simulink model "Application_Problem_Solution"  (R2018b)
settings: Solver=VariableStepAuto  StartTime=0.0  StopTime=6300  FixedStep=0.1  RelTol=1e-3  EnableMultiTasking=on
StopFcn:
  | if sum(Diagnostic_Decision_PV_1)>0
  | f = msgbox('Failure in PV 1');
  | end
  | 
  | if sum(Diagnostic_Decision_PV_2)>0
  | f = msgbox('Failure in PV 2');
  | end
  | 
  | if sum(Diagnostic_Decision_PV_3)>0
  | f = msgbox('Failure in PV 3');
  | end
  | 
  | if sum(Diagnostic_Decision_PV_4)>0
  | f = msgbox('Failure in PV 4');
  | end
  | 
  | if sum(Diagnostic_Decision_PV_5)>0
  | f = msgbox('Failure in PV 5');
  | end
  | 
  | if sum(Diagnostic_Decision_PV_6)>0
  | f = msgbox('Failure in PV 6');
  | end
  | 
  | if sum(Diagnostic_Decision_PV_7)>0
  | f = msgbox('Failure in PV 7');
  | end
  | 
  | if sum(Diagnostic_Decision_PV_8)>0
  | f = msgbox('Failure in PV 8');
  | end
  | 
  | if sum(Diagnostic_Decision_PV_9)>0
  | f = msgbox('Failure in PV 9');
  | end
  | 
  | if sum(Diagnostic_Decision_PV_10)>0
  | f = msgbox('Failure in PV 10');
  | end
values from neighbouring files (symbols this model uses):
  C1_LUT = [1913.6 4625.7 23306 10736 18036 12251 9022.9 12447 18872 40764 18721 33630 ... (21 elements, 7x3)]    [model_data_application.mat]
  Capacity_LUT = [28.0081 27.625 27.6392]    [model_data_application.mat]
  cell_Cp_heat = 810.5328    [model_data_application.mat]
  cell_mass = 1    [model_data_application.mat]
  Em_LUT = [3.4966 3.5519 3.6183 3.7066 3.9131 4.0748 4.1923 3.5057 3.566 3.6337 3.7127 3.9259 ... (21 elements, 7x3)]    [model_data_application.mat]
  Qe_init = 3.6845    [model_data_application.mat]
  R0_LUT = [0.0117 0.011 0.0114 0.0107 0.0107 0.0113 0.0116 0.0085 0.0085 0.0087 0.0082 0.0083 ... (21 elements, 7x3)]    [model_data_application.mat]
  R1_LUT = [0.0109 0.0069 0.0047 0.0034 0.0033 0.0033 0.0028 0.0029 0.0024 0.0026 0.0016 0.0023 ... (21 elements, 7x3)]    [model_data_application.mat]
  SOC_LUT = [0 0.1 0.25 0.5 0.75 0.9 1]    [model_data_application.mat]
  T_init = 293.15    [model_data_application.mat]
  Temperature_LUT = [278.15 293.15 313.15]    [model_data_application.mat]
undefined symbols (not defined in the file or in its folder): DiscIntNeverNeededParam
libraries: elec_lib x450, fl_lib x121, LiBatteryElements_lib x40, nesl_utility x32, simulink x10
(part 3 of 3)

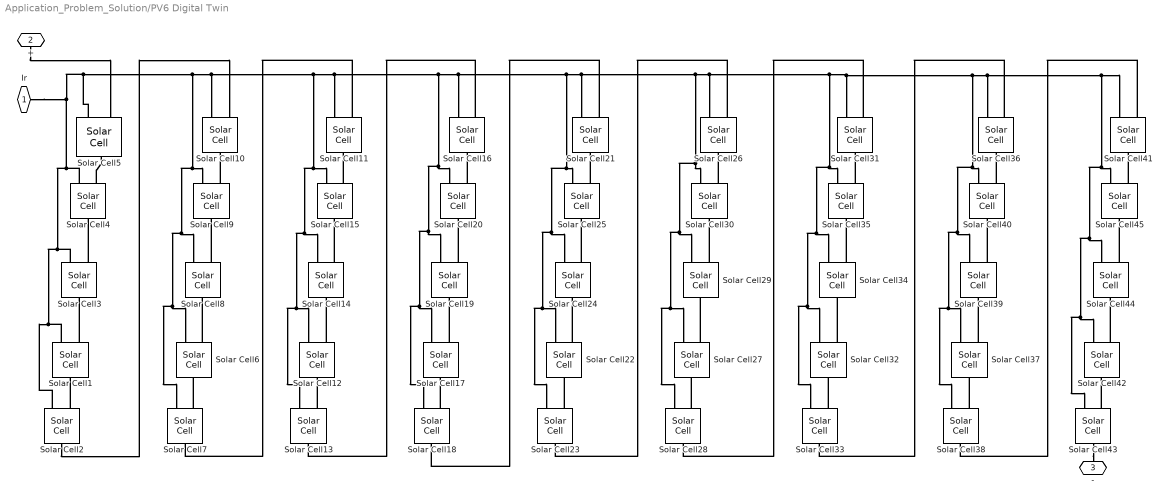
== system Application_Problem_Solution/PV6 Digital Twin ==
  Solar Cell{1..45} (45 alike) : elec_lib/Sources/Solar Cell  prm=1  Isc=Isc A  Voc=Voc/45 V  Is=1e-6 A  Is2=0 A  Iph=7.34 A  Ir0=Ir0 W/m^2  ec=n  N2=2  Rs=Rs/45 Ohm  Rp=Inf Ohm  N_series=1  TIPH1=0 1/K  EG=1.11 eV  TXIS1=3  TXIS2=3  TRS1=0  TRP1=0  Tmeas=T degC  TFIXED=T degC  thermal_mass=100 J/K  initial_temperature=25 degC
      settings: SourceProductName=Simscape Electronics  SourceProductBaseCode=SN
  Ir : PMIOPort  Side=Left
  + : PMIOPort  Port=2  Side=Right
  - : PMIOPort  Port=3  Side=Right
  connections:
  Solar Cell43/RConn1 -- -/RConn1
  Solar Cell43/LConn2 -- Solar Cell42/RConn1
  Solar Cell42/LConn2 -- Solar Cell44/RConn1
  Solar Cell45/LConn2 -- Solar Cell41/RConn1
  Solar Cell41/LConn2 -- Solar Cell38/RConn1
  Solar Cell44/LConn2 -- Solar Cell45/RConn1
  Solar Cell38/LConn2 -- Solar Cell37/RConn1
  Solar Cell37/LConn2 -- Solar Cell39/RConn1
  Solar Cell40/LConn2 -- Solar Cell36/RConn1
  Solar Cell36/LConn2 -- Solar Cell33/RConn1
  Solar Cell39/LConn2 -- Solar Cell40/RConn1
  Solar Cell33/LConn2 -- Solar Cell32/RConn1
  Solar Cell32/LConn2 -- Solar Cell34/RConn1
  Solar Cell35/LConn2 -- Solar Cell31/RConn1
  Solar Cell31/LConn2 -- Solar Cell28/RConn1
  Solar Cell34/LConn2 -- Solar Cell35/RConn1
  Solar Cell28/LConn2 -- Solar Cell27/RConn1
  Solar Cell27/LConn2 -- Solar Cell29/RConn1
  Solar Cell30/LConn2 -- Solar Cell26/RConn1
  Solar Cell26/LConn2 -- Solar Cell23/RConn1
  Solar Cell29/LConn2 -- Solar Cell30/RConn1
  Solar Cell24/LConn2 -- Solar Cell25/RConn1
  Solar Cell21/LConn2 -- Solar Cell18/RConn1
  Solar Cell25/LConn2 -- Solar Cell21/RConn1
  Solar Cell22/LConn2 -- Solar Cell24/RConn1
  Solar Cell23/LConn2 -- Solar Cell22/RConn1
  Solar Cell18/LConn2 -- Solar Cell17/RConn1
  Solar Cell17/LConn2 -- Solar Cell19/RConn1
  Solar Cell16/LConn2 -- Solar Cell13/RConn1
  Solar Cell20/LConn2 -- Solar Cell16/RConn1
  Solar Cell19/LConn2 -- Solar Cell20/RConn1
  Solar Cell14/LConn2 -- Solar Cell15/RConn1
  Solar Cell15/LConn2 -- Solar Cell11/RConn1
  Solar Cell13/LConn2 -- Solar Cell12/RConn1
  Solar Cell12/LConn2 -- Solar Cell14/RConn1
  Solar Cell11/LConn2 -- Solar Cell7/RConn1
  Solar Cell8/LConn2 -- Solar Cell9/RConn1
  Solar Cell2/RConn1 -- Solar Cell10/LConn2
  Solar Cell6/LConn2 -- Solar Cell8/RConn1
  Solar Cell7/LConn2 -- Solar Cell6/RConn1
  Solar Cell9/LConn2 -- Solar Cell10/RConn1
  +/RConn1 -- Solar Cell5/LConn2
  Solar Cell4/LConn2 -- Solar Cell5/RConn1
  Solar Cell1/LConn2 -- Solar Cell3/RConn1
  Solar Cell2/LConn2 -- Solar Cell1/RConn1
  Solar Cell3/LConn2 -- Solar Cell4/RConn1
  Ir/RConn1 -- Solar Cell2/LConn1 -- Solar Cell1/LConn1 -- Solar Cell3/LConn1 -- Solar Cell4/LConn1 -- Solar Cell10/LConn1 -- Solar Cell11/LConn1 -- Solar Cell16/LConn1 -- Solar Cell21/LConn1 -- Solar Cell26/LConn1 -- Solar Cell31/LConn1 -- Solar Cell36/LConn1 -- Solar Cell41/LConn1 -- Solar Cell45/LConn1 -- Solar Cell44/LConn1 -- Solar Cell42/LConn1 -- Solar Cell43/LConn1 -- Solar Cell40/LConn1 -- Solar Cell39/LConn1 -- Solar Cell38/LConn1 -- Solar Cell37/LConn1 -- Solar Cell35/LConn1 -- Solar Cell34/LConn1 -- Solar Cell32/LConn1 -- Solar Cell33/LConn1 -- Solar Cell30/LConn1 -- Solar Cell29/LConn1 -- Solar Cell27/LConn1 -- Solar Cell28/LConn1 -- Solar Cell25/LConn1 -- Solar Cell24/LConn1 -- Solar Cell23/LConn1 -- Solar Cell22/LConn1 -- Solar Cell20/LConn1 -- Solar Cell19/LConn1 -- Solar Cell17/LConn1 -- Solar Cell18/LConn1 -- Solar Cell15/LConn1 -- Solar Cell14/LConn1 -- Solar Cell12/LConn1 -- Solar Cell13/LConn1 -- Solar Cell9/LConn1 -- Solar Cell8/LConn1 -- Solar Cell6/LConn1 -- Solar Cell7/LConn1 -- Solar Cell5/LConn1

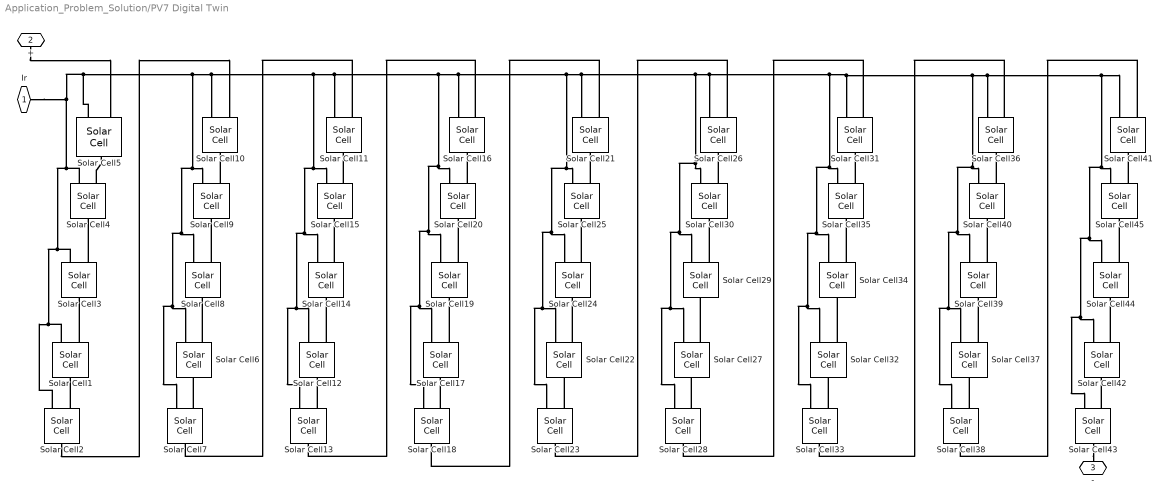
== system Application_Problem_Solution/PV7 Digital Twin ==
  Solar Cell{1..45} (45 alike) : elec_lib/Sources/Solar Cell  prm=1  Isc=Isc A  Voc=Voc/45 V  Is=1e-6 A  Is2=0 A  Iph=7.34 A  Ir0=Ir0 W/m^2  ec=n  N2=2  Rs=Rs/45 Ohm  Rp=Inf Ohm  N_series=1  TIPH1=0 1/K  EG=1.11 eV  TXIS1=3  TXIS2=3  TRS1=0  TRP1=0  Tmeas=T degC  TFIXED=T degC  thermal_mass=100 J/K  initial_temperature=25 degC
      settings: SourceProductName=Simscape Electronics  SourceProductBaseCode=SN
  Ir : PMIOPort  Side=Left
  + : PMIOPort  Port=2  Side=Right
  - : PMIOPort  Port=3  Side=Right
  connections:
  Solar Cell5/LConn1 -- Solar Cell7/LConn1 -- Solar Cell6/LConn1 -- Solar Cell8/LConn1 -- Solar Cell9/LConn1 -- Solar Cell13/LConn1 -- Solar Cell12/LConn1 -- Solar Cell14/LConn1 -- Solar Cell15/LConn1 -- Solar Cell18/LConn1 -- Solar Cell17/LConn1 -- Solar Cell19/LConn1 -- Solar Cell20/LConn1 -- Solar Cell22/LConn1 -- Solar Cell23/LConn1 -- Solar Cell24/LConn1 -- Solar Cell25/LConn1 -- Solar Cell28/LConn1 -- Solar Cell27/LConn1 -- Solar Cell29/LConn1 -- Solar Cell30/LConn1 -- Solar Cell33/LConn1 -- Solar Cell32/LConn1 -- Solar Cell34/LConn1 -- Solar Cell35/LConn1 -- Solar Cell37/LConn1 -- Solar Cell38/LConn1 -- Solar Cell39/LConn1 -- Solar Cell40/LConn1 -- Solar Cell43/LConn1 -- Solar Cell42/LConn1 -- Solar Cell44/LConn1 -- Solar Cell45/LConn1 -- Solar Cell41/LConn1 -- Solar Cell36/LConn1 -- Solar Cell31/LConn1 -- Solar Cell26/LConn1 -- Solar Cell21/LConn1 -- Solar Cell16/LConn1 -- Solar Cell11/LConn1 -- Solar Cell10/LConn1 -- Solar Cell4/LConn1 -- Solar Cell3/LConn1 -- Solar Cell1/LConn1 -- Solar Cell2/LConn1 -- Ir/RConn1
  Solar Cell3/LConn2 -- Solar Cell4/RConn1
  Solar Cell2/LConn2 -- Solar Cell1/RConn1
  Solar Cell1/LConn2 -- Solar Cell3/RConn1
  Solar Cell4/LConn2 -- Solar Cell5/RConn1
  +/RConn1 -- Solar Cell5/LConn2
  Solar Cell9/LConn2 -- Solar Cell10/RConn1
  Solar Cell7/LConn2 -- Solar Cell6/RConn1
  Solar Cell6/LConn2 -- Solar Cell8/RConn1
  Solar Cell2/RConn1 -- Solar Cell10/LConn2
  Solar Cell8/LConn2 -- Solar Cell9/RConn1
  Solar Cell11/LConn2 -- Solar Cell7/RConn1
  Solar Cell12/LConn2 -- Solar Cell14/RConn1
  Solar Cell13/LConn2 -- Solar Cell12/RConn1
  Solar Cell15/LConn2 -- Solar Cell11/RConn1
  Solar Cell14/LConn2 -- Solar Cell15/RConn1
  Solar Cell19/LConn2 -- Solar Cell20/RConn1
  Solar Cell20/LConn2 -- Solar Cell16/RConn1
  Solar Cell16/LConn2 -- Solar Cell13/RConn1
  Solar Cell17/LConn2 -- Solar Cell19/RConn1
  Solar Cell18/LConn2 -- Solar Cell17/RConn1
  Solar Cell23/LConn2 -- Solar Cell22/RConn1
  Solar Cell22/LConn2 -- Solar Cell24/RConn1
  Solar Cell25/LConn2 -- Solar Cell21/RConn1
  Solar Cell21/LConn2 -- Solar Cell18/RConn1
  Solar Cell24/LConn2 -- Solar Cell25/RConn1
  Solar Cell29/LConn2 -- Solar Cell30/RConn1
  Solar Cell26/LConn2 -- Solar Cell23/RConn1
  Solar Cell30/LConn2 -- Solar Cell26/RConn1
  Solar Cell27/LConn2 -- Solar Cell29/RConn1
  Solar Cell28/LConn2 -- Solar Cell27/RConn1
  Solar Cell34/LConn2 -- Solar Cell35/RConn1
  Solar Cell31/LConn2 -- Solar Cell28/RConn1
  Solar Cell35/LConn2 -- Solar Cell31/RConn1
  Solar Cell32/LConn2 -- Solar Cell34/RConn1
  Solar Cell33/LConn2 -- Solar Cell32/RConn1
  Solar Cell39/LConn2 -- Solar Cell40/RConn1
  Solar Cell36/LConn2 -- Solar Cell33/RConn1
  Solar Cell40/LConn2 -- Solar Cell36/RConn1
  Solar Cell37/LConn2 -- Solar Cell39/RConn1
  Solar Cell38/LConn2 -- Solar Cell37/RConn1
  Solar Cell44/LConn2 -- Solar Cell45/RConn1
  Solar Cell41/LConn2 -- Solar Cell38/RConn1
  Solar Cell45/LConn2 -- Solar Cell41/RConn1
  Solar Cell42/LConn2 -- Solar Cell44/RConn1
  Solar Cell43/LConn2 -- Solar Cell42/RConn1
  Solar Cell43/RConn1 -- -/RConn1

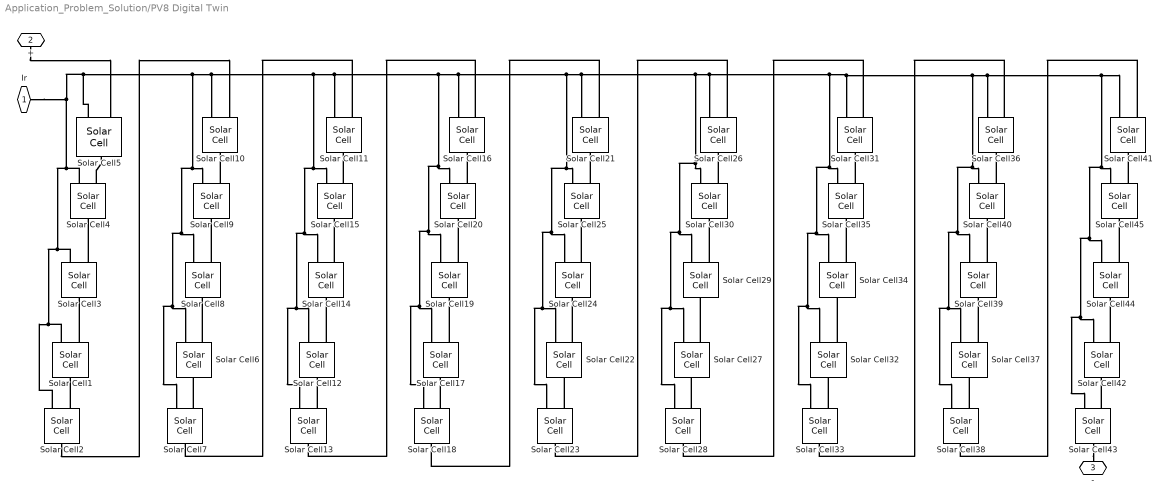
== system Application_Problem_Solution/PV8 Digital Twin ==
  Solar Cell{1..45} (45 alike) : elec_lib/Sources/Solar Cell  prm=1  Isc=Isc A  Voc=Voc/45 V  Is=1e-6 A  Is2=0 A  Iph=7.34 A  Ir0=Ir0 W/m^2  ec=n  N2=2  Rs=Rs/45 Ohm  Rp=Inf Ohm  N_series=1  TIPH1=0 1/K  EG=1.11 eV  TXIS1=3  TXIS2=3  TRS1=0  TRP1=0  Tmeas=T degC  TFIXED=T degC  thermal_mass=100 J/K  initial_temperature=25 degC
      settings: SourceProductName=Simscape Electronics  SourceProductBaseCode=SN
  Ir : PMIOPort  Side=Left
  + : PMIOPort  Port=2  Side=Right
  - : PMIOPort  Port=3  Side=Right
  connections:
  Solar Cell43/RConn1 -- -/RConn1
  Solar Cell43/LConn2 -- Solar Cell42/RConn1
  Solar Cell42/LConn2 -- Solar Cell44/RConn1
  Solar Cell45/LConn2 -- Solar Cell41/RConn1
  Solar Cell41/LConn2 -- Solar Cell38/RConn1
  Solar Cell44/LConn2 -- Solar Cell45/RConn1
  Solar Cell38/LConn2 -- Solar Cell37/RConn1
  Solar Cell37/LConn2 -- Solar Cell39/RConn1
  Solar Cell40/LConn2 -- Solar Cell36/RConn1
  Solar Cell36/LConn2 -- Solar Cell33/RConn1
  Solar Cell39/LConn2 -- Solar Cell40/RConn1
  Solar Cell33/LConn2 -- Solar Cell32/RConn1
  Solar Cell32/LConn2 -- Solar Cell34/RConn1
  Solar Cell35/LConn2 -- Solar Cell31/RConn1
  Solar Cell31/LConn2 -- Solar Cell28/RConn1
  Solar Cell34/LConn2 -- Solar Cell35/RConn1
  Solar Cell28/LConn2 -- Solar Cell27/RConn1
  Solar Cell27/LConn2 -- Solar Cell29/RConn1
  Solar Cell30/LConn2 -- Solar Cell26/RConn1
  Solar Cell26/LConn2 -- Solar Cell23/RConn1
  Solar Cell29/LConn2 -- Solar Cell30/RConn1
  Solar Cell24/LConn2 -- Solar Cell25/RConn1
  Solar Cell21/LConn2 -- Solar Cell18/RConn1
  Solar Cell25/LConn2 -- Solar Cell21/RConn1
  Solar Cell22/LConn2 -- Solar Cell24/RConn1
  Solar Cell23/LConn2 -- Solar Cell22/RConn1
  Solar Cell18/LConn2 -- Solar Cell17/RConn1
  Solar Cell17/LConn2 -- Solar Cell19/RConn1
  Solar Cell16/LConn2 -- Solar Cell13/RConn1
  Solar Cell20/LConn2 -- Solar Cell16/RConn1
  Solar Cell19/LConn2 -- Solar Cell20/RConn1
  Solar Cell14/LConn2 -- Solar Cell15/RConn1
  Solar Cell15/LConn2 -- Solar Cell11/RConn1
  Solar Cell13/LConn2 -- Solar Cell12/RConn1
  Solar Cell12/LConn2 -- Solar Cell14/RConn1
  Solar Cell11/LConn2 -- Solar Cell7/RConn1
  Solar Cell8/LConn2 -- Solar Cell9/RConn1
  Solar Cell2/RConn1 -- Solar Cell10/LConn2
  Solar Cell6/LConn2 -- Solar Cell8/RConn1
  Solar Cell7/LConn2 -- Solar Cell6/RConn1
  Solar Cell9/LConn2 -- Solar Cell10/RConn1
  +/RConn1 -- Solar Cell5/LConn2
  Solar Cell4/LConn2 -- Solar Cell5/RConn1
  Solar Cell1/LConn2 -- Solar Cell3/RConn1
  Solar Cell2/LConn2 -- Solar Cell1/RConn1
  Solar Cell3/LConn2 -- Solar Cell4/RConn1
  Ir/RConn1 -- Solar Cell2/LConn1 -- Solar Cell1/LConn1 -- Solar Cell3/LConn1 -- Solar Cell4/LConn1 -- Solar Cell10/LConn1 -- Solar Cell11/LConn1 -- Solar Cell16/LConn1 -- Solar Cell21/LConn1 -- Solar Cell26/LConn1 -- Solar Cell31/LConn1 -- Solar Cell36/LConn1 -- Solar Cell41/LConn1 -- Solar Cell45/LConn1 -- Solar Cell44/LConn1 -- Solar Cell42/LConn1 -- Solar Cell43/LConn1 -- Solar Cell40/LConn1 -- Solar Cell39/LConn1 -- Solar Cell38/LConn1 -- Solar Cell37/LConn1 -- Solar Cell35/LConn1 -- Solar Cell34/LConn1 -- Solar Cell32/LConn1 -- Solar Cell33/LConn1 -- Solar Cell30/LConn1 -- Solar Cell29/LConn1 -- Solar Cell27/LConn1 -- Solar Cell28/LConn1 -- Solar Cell25/LConn1 -- Solar Cell24/LConn1 -- Solar Cell23/LConn1 -- Solar Cell22/LConn1 -- Solar Cell20/LConn1 -- Solar Cell19/LConn1 -- Solar Cell17/LConn1 -- Solar Cell18/LConn1 -- Solar Cell15/LConn1 -- Solar Cell14/LConn1 -- Solar Cell12/LConn1 -- Solar Cell13/LConn1 -- Solar Cell9/LConn1 -- Solar Cell8/LConn1 -- Solar Cell6/LConn1 -- Solar Cell7/LConn1 -- Solar Cell5/LConn1

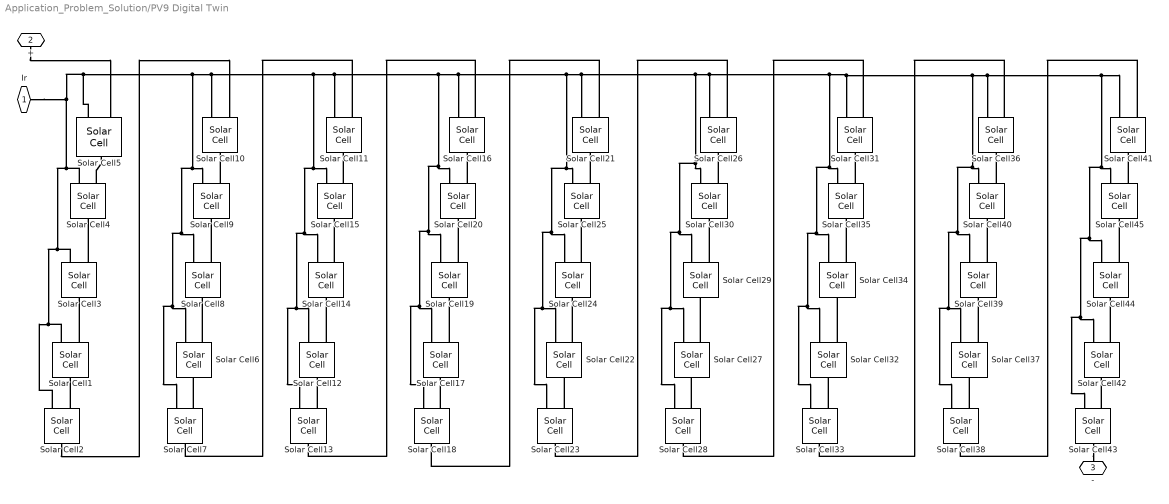
== system Application_Problem_Solution/PV9 Digital Twin ==
  Solar Cell{1..45} (45 alike) : elec_lib/Sources/Solar Cell  prm=1  Isc=Isc A  Voc=Voc/45 V  Is=1e-6 A  Is2=0 A  Iph=7.34 A  Ir0=Ir0 W/m^2  ec=n  N2=2  Rs=Rs/45 Ohm  Rp=Inf Ohm  N_series=1  TIPH1=0 1/K  EG=1.11 eV  TXIS1=3  TXIS2=3  TRS1=0  TRP1=0  Tmeas=T degC  TFIXED=T degC  thermal_mass=100 J/K  initial_temperature=25 degC
      settings: SourceProductName=Simscape Electronics  SourceProductBaseCode=SN
  Ir : PMIOPort  Side=Left
  + : PMIOPort  Port=2  Side=Right
  - : PMIOPort  Port=3  Side=Right
  connections:
  Solar Cell5/LConn1 -- Solar Cell7/LConn1 -- Solar Cell6/LConn1 -- Solar Cell8/LConn1 -- Solar Cell9/LConn1 -- Solar Cell13/LConn1 -- Solar Cell12/LConn1 -- Solar Cell14/LConn1 -- Solar Cell15/LConn1 -- Solar Cell18/LConn1 -- Solar Cell17/LConn1 -- Solar Cell19/LConn1 -- Solar Cell20/LConn1 -- Solar Cell22/LConn1 -- Solar Cell23/LConn1 -- Solar Cell24/LConn1 -- Solar Cell25/LConn1 -- Solar Cell28/LConn1 -- Solar Cell27/LConn1 -- Solar Cell29/LConn1 -- Solar Cell30/LConn1 -- Solar Cell33/LConn1 -- Solar Cell32/LConn1 -- Solar Cell34/LConn1 -- Solar Cell35/LConn1 -- Solar Cell37/LConn1 -- Solar Cell38/LConn1 -- Solar Cell39/LConn1 -- Solar Cell40/LConn1 -- Solar Cell43/LConn1 -- Solar Cell42/LConn1 -- Solar Cell44/LConn1 -- Solar Cell45/LConn1 -- Solar Cell41/LConn1 -- Solar Cell36/LConn1 -- Solar Cell31/LConn1 -- Solar Cell26/LConn1 -- Solar Cell21/LConn1 -- Solar Cell16/LConn1 -- Solar Cell11/LConn1 -- Solar Cell10/LConn1 -- Solar Cell4/LConn1 -- Solar Cell3/LConn1 -- Solar Cell1/LConn1 -- Solar Cell2/LConn1 -- Ir/RConn1
  Solar Cell3/LConn2 -- Solar Cell4/RConn1
  Solar Cell2/LConn2 -- Solar Cell1/RConn1
  Solar Cell1/LConn2 -- Solar Cell3/RConn1
  Solar Cell4/LConn2 -- Solar Cell5/RConn1
  +/RConn1 -- Solar Cell5/LConn2
  Solar Cell9/LConn2 -- Solar Cell10/RConn1
  Solar Cell7/LConn2 -- Solar Cell6/RConn1
  Solar Cell6/LConn2 -- Solar Cell8/RConn1
  Solar Cell2/RConn1 -- Solar Cell10/LConn2
  Solar Cell8/LConn2 -- Solar Cell9/RConn1
  Solar Cell11/LConn2 -- Solar Cell7/RConn1
  Solar Cell12/LConn2 -- Solar Cell14/RConn1
  Solar Cell13/LConn2 -- Solar Cell12/RConn1
  Solar Cell15/LConn2 -- Solar Cell11/RConn1
  Solar Cell14/LConn2 -- Solar Cell15/RConn1
  Solar Cell19/LConn2 -- Solar Cell20/RConn1
  Solar Cell20/LConn2 -- Solar Cell16/RConn1
  Solar Cell16/LConn2 -- Solar Cell13/RConn1
  Solar Cell17/LConn2 -- Solar Cell19/RConn1
  Solar Cell18/LConn2 -- Solar Cell17/RConn1
  Solar Cell23/LConn2 -- Solar Cell22/RConn1
  Solar Cell22/LConn2 -- Solar Cell24/RConn1
  Solar Cell25/LConn2 -- Solar Cell21/RConn1
  Solar Cell21/LConn2 -- Solar Cell18/RConn1
  Solar Cell24/LConn2 -- Solar Cell25/RConn1
  Solar Cell29/LConn2 -- Solar Cell30/RConn1
  Solar Cell26/LConn2 -- Solar Cell23/RConn1
  Solar Cell30/LConn2 -- Solar Cell26/RConn1
  Solar Cell27/LConn2 -- Solar Cell29/RConn1
  Solar Cell28/LConn2 -- Solar Cell27/RConn1
  Solar Cell34/LConn2 -- Solar Cell35/RConn1
  Solar Cell31/LConn2 -- Solar Cell28/RConn1
  Solar Cell35/LConn2 -- Solar Cell31/RConn1
  Solar Cell32/LConn2 -- Solar Cell34/RConn1
  Solar Cell33/LConn2 -- Solar Cell32/RConn1
  Solar Cell39/LConn2 -- Solar Cell40/RConn1
  Solar Cell36/LConn2 -- Solar Cell33/RConn1
  Solar Cell40/LConn2 -- Solar Cell36/RConn1
  Solar Cell37/LConn2 -- Solar Cell39/RConn1
  Solar Cell38/LConn2 -- Solar Cell37/RConn1
  Solar Cell44/LConn2 -- Solar Cell45/RConn1
  Solar Cell41/LConn2 -- Solar Cell38/RConn1
  Solar Cell45/LConn2 -- Solar Cell41/RConn1
  Solar Cell42/LConn2 -- Solar Cell44/RConn1
  Solar Cell43/LConn2 -- Solar Cell42/RConn1
  Solar Cell43/RConn1 -- -/RConn1

== system Application_Problem_Solution/Battery1/Thermal Model ==
  Battery thermal mass : fl_lib/Thermal/Thermal Elements/Thermal Mass  mass=cell_mass kg  sp_heat=cell_Cp_heat J/kg/K  T_specify=on  T_priority=High  T=T_init K  T_nominal_specify=off  T_nominal_unit=K  T_nominal_value=1  Q_specify=off  Q_priority=High  Q=0 J/s  Q_nominal_specify=off  Q_nominal_unit=W  Q_nominal_value=1
  Ideal Temperature Sensor : fl_lib/Thermal/Thermal Sensors/Temperature Sensor
  Ideal Heat Flow Source : fl_lib/Thermal/Thermal Sources/Controlled Heat Flow Rate Source
      settings: SourceProductName=Simscape
  Thermal Reference1 : fl_lib/Thermal/Thermal Elements/Thermal Reference
  Thermal Reference2 : fl_lib/Thermal/Thermal Elements/Thermal Reference
  P_in : PMIOPort  Tag=PMCPort  Side=Left
  H : PMIOPort  Tag=PMCPort  Port=2  Side=Left
  T : PMIOPort  Tag=PMCPort  Port=3  Side=Right
  connections:
  Thermal Reference2/LConn1 -- Ideal Temperature Sensor/RConn1
  Ideal Temperature Sensor/RConn2 -- T/RConn1
  Thermal Reference1/LConn1 -- Ideal Heat Flow Source/RConn2
  Ideal Temperature Sensor/LConn1 -- H/RConn1 -- Battery thermal mass/LConn1 -- Ideal Heat Flow Source/LConn1
  Ideal Heat Flow Source/RConn1 -- P_in/RConn1

== system Application_Problem_Solution/Battery10/Thermal Model ==
  Battery thermal mass : fl_lib/Thermal/Thermal Elements/Thermal Mass  mass=cell_mass kg  sp_heat=cell_Cp_heat J/kg/K  T_specify=on  T_priority=High  T=T_init K  T_nominal_specify=off  T_nominal_unit=K  T_nominal_value=1  Q_specify=off  Q_priority=High  Q=0 J/s  Q_nominal_specify=off  Q_nominal_unit=W  Q_nominal_value=1
  Ideal Temperature Sensor : fl_lib/Thermal/Thermal Sensors/Temperature Sensor
  Ideal Heat Flow Source : fl_lib/Thermal/Thermal Sources/Controlled Heat Flow Rate Source
      settings: SourceProductName=Simscape
  Thermal Reference1 : fl_lib/Thermal/Thermal Elements/Thermal Reference
  Thermal Reference2 : fl_lib/Thermal/Thermal Elements/Thermal Reference
  P_in : PMIOPort  Tag=PMCPort  Side=Left
  H : PMIOPort  Tag=PMCPort  Port=2  Side=Left
  T : PMIOPort  Tag=PMCPort  Port=3  Side=Right
  connections:
  Thermal Reference2/LConn1 -- Ideal Temperature Sensor/RConn1
  Ideal Temperature Sensor/RConn2 -- T/RConn1
  Thermal Reference1/LConn1 -- Ideal Heat Flow Source/RConn2
  Ideal Temperature Sensor/LConn1 -- H/RConn1 -- Battery thermal mass/LConn1 -- Ideal Heat Flow Source/LConn1
  Ideal Heat Flow Source/RConn1 -- P_in/RConn1

== system Application_Problem_Solution/Battery2/Thermal Model ==
  Battery thermal mass : fl_lib/Thermal/Thermal Elements/Thermal Mass  mass=cell_mass kg  sp_heat=cell_Cp_heat J/kg/K  T_specify=on  T_priority=High  T=T_init K  T_nominal_specify=off  T_nominal_unit=K  T_nominal_value=1  Q_specify=off  Q_priority=High  Q=0 J/s  Q_nominal_specify=off  Q_nominal_unit=W  Q_nominal_value=1
  Ideal Temperature Sensor : fl_lib/Thermal/Thermal Sensors/Temperature Sensor
  Ideal Heat Flow Source : fl_lib/Thermal/Thermal Sources/Controlled Heat Flow Rate Source
      settings: SourceProductName=Simscape
  Thermal Reference1 : fl_lib/Thermal/Thermal Elements/Thermal Reference
  Thermal Reference2 : fl_lib/Thermal/Thermal Elements/Thermal Reference
  P_in : PMIOPort  Tag=PMCPort  Side=Left
  H : PMIOPort  Tag=PMCPort  Port=2  Side=Left
  T : PMIOPort  Tag=PMCPort  Port=3  Side=Right
  connections:
  Thermal Reference2/LConn1 -- Ideal Temperature Sensor/RConn1
  Ideal Temperature Sensor/RConn2 -- T/RConn1
  Thermal Reference1/LConn1 -- Ideal Heat Flow Source/RConn2
  Ideal Temperature Sensor/LConn1 -- H/RConn1 -- Battery thermal mass/LConn1 -- Ideal Heat Flow Source/LConn1
  Ideal Heat Flow Source/RConn1 -- P_in/RConn1

== system Application_Problem_Solution/Battery3/Thermal Model ==
  Battery thermal mass : fl_lib/Thermal/Thermal Elements/Thermal Mass  mass=cell_mass kg  sp_heat=cell_Cp_heat J/kg/K  T_specify=on  T_priority=High  T=T_init K  T_nominal_specify=off  T_nominal_unit=K  T_nominal_value=1  Q_specify=off  Q_priority=High  Q=0 J/s  Q_nominal_specify=off  Q_nominal_unit=W  Q_nominal_value=1
  Ideal Temperature Sensor : fl_lib/Thermal/Thermal Sensors/Temperature Sensor
  Ideal Heat Flow Source : fl_lib/Thermal/Thermal Sources/Controlled Heat Flow Rate Source
      settings: SourceProductName=Simscape
  Thermal Reference1 : fl_lib/Thermal/Thermal Elements/Thermal Reference
  Thermal Reference2 : fl_lib/Thermal/Thermal Elements/Thermal Reference
  P_in : PMIOPort  Tag=PMCPort  Side=Left
  H : PMIOPort  Tag=PMCPort  Port=2  Side=Left
  T : PMIOPort  Tag=PMCPort  Port=3  Side=Right
  connections:
  Ideal Heat Flow Source/RConn1 -- P_in/RConn1
  Ideal Heat Flow Source/LConn1 -- Battery thermal mass/LConn1 -- H/RConn1 -- Ideal Temperature Sensor/LConn1
  Thermal Reference1/LConn1 -- Ideal Heat Flow Source/RConn2
  Ideal Temperature Sensor/RConn2 -- T/RConn1
  Thermal Reference2/LConn1 -- Ideal Temperature Sensor/RConn1

== system Application_Problem_Solution/Battery4/Thermal Model ==
  Battery thermal mass : fl_lib/Thermal/Thermal Elements/Thermal Mass  mass=cell_mass kg  sp_heat=cell_Cp_heat J/kg/K  T_specify=on  T_priority=High  T=T_init K  T_nominal_specify=off  T_nominal_unit=K  T_nominal_value=1  Q_specify=off  Q_priority=High  Q=0 J/s  Q_nominal_specify=off  Q_nominal_unit=W  Q_nominal_value=1
  Ideal Temperature Sensor : fl_lib/Thermal/Thermal Sensors/Temperature Sensor
  Ideal Heat Flow Source : fl_lib/Thermal/Thermal Sources/Controlled Heat Flow Rate Source
      settings: SourceProductName=Simscape
  Thermal Reference1 : fl_lib/Thermal/Thermal Elements/Thermal Reference
  Thermal Reference2 : fl_lib/Thermal/Thermal Elements/Thermal Reference
  P_in : PMIOPort  Tag=PMCPort  Side=Left
  H : PMIOPort  Tag=PMCPort  Port=2  Side=Left
  T : PMIOPort  Tag=PMCPort  Port=3  Side=Right
  connections:
  Thermal Reference2/LConn1 -- Ideal Temperature Sensor/RConn1
  Ideal Temperature Sensor/RConn2 -- T/RConn1
  Thermal Reference1/LConn1 -- Ideal Heat Flow Source/RConn2
  Ideal Temperature Sensor/LConn1 -- H/RConn1 -- Battery thermal mass/LConn1 -- Ideal Heat Flow Source/LConn1
  Ideal Heat Flow Source/RConn1 -- P_in/RConn1

== system Application_Problem_Solution/Battery5/Thermal Model ==
  Battery thermal mass : fl_lib/Thermal/Thermal Elements/Thermal Mass  mass=cell_mass kg  sp_heat=cell_Cp_heat J/kg/K  T_specify=on  T_priority=High  T=T_init K  T_nominal_specify=off  T_nominal_unit=K  T_nominal_value=1  Q_specify=off  Q_priority=High  Q=0 J/s  Q_nominal_specify=off  Q_nominal_unit=W  Q_nominal_value=1
  Ideal Temperature Sensor : fl_lib/Thermal/Thermal Sensors/Temperature Sensor
  Ideal Heat Flow Source : fl_lib/Thermal/Thermal Sources/Controlled Heat Flow Rate Source
      settings: SourceProductName=Simscape
  Thermal Reference1 : fl_lib/Thermal/Thermal Elements/Thermal Reference
  Thermal Reference2 : fl_lib/Thermal/Thermal Elements/Thermal Reference
  P_in : PMIOPort  Tag=PMCPort  Side=Left
  H : PMIOPort  Tag=PMCPort  Port=2  Side=Left
  T : PMIOPort  Tag=PMCPort  Port=3  Side=Right
  connections:
  Ideal Heat Flow Source/RConn1 -- P_in/RConn1
  Ideal Heat Flow Source/LConn1 -- Battery thermal mass/LConn1 -- H/RConn1 -- Ideal Temperature Sensor/LConn1
  Thermal Reference1/LConn1 -- Ideal Heat Flow Source/RConn2
  Ideal Temperature Sensor/RConn2 -- T/RConn1
  Thermal Reference2/LConn1 -- Ideal Temperature Sensor/RConn1

== system Application_Problem_Solution/Battery6/Thermal Model ==
  Battery thermal mass : fl_lib/Thermal/Thermal Elements/Thermal Mass  mass=cell_mass kg  sp_heat=cell_Cp_heat J/kg/K  T_specify=on  T_priority=High  T=T_init K  T_nominal_specify=off  T_nominal_unit=K  T_nominal_value=1  Q_specify=off  Q_priority=High  Q=0 J/s  Q_nominal_specify=off  Q_nominal_unit=W  Q_nominal_value=1
  Ideal Temperature Sensor : fl_lib/Thermal/Thermal Sensors/Temperature Sensor
  Ideal Heat Flow Source : fl_lib/Thermal/Thermal Sources/Controlled Heat Flow Rate Source
      settings: SourceProductName=Simscape
  Thermal Reference1 : fl_lib/Thermal/Thermal Elements/Thermal Reference
  Thermal Reference2 : fl_lib/Thermal/Thermal Elements/Thermal Reference
  P_in : PMIOPort  Tag=PMCPort  Side=Left
  H : PMIOPort  Tag=PMCPort  Port=2  Side=Left
  T : PMIOPort  Tag=PMCPort  Port=3  Side=Right
  connections:
  Thermal Reference2/LConn1 -- Ideal Temperature Sensor/RConn1
  Ideal Temperature Sensor/RConn2 -- T/RConn1
  Thermal Reference1/LConn1 -- Ideal Heat Flow Source/RConn2
  Ideal Temperature Sensor/LConn1 -- H/RConn1 -- Battery thermal mass/LConn1 -- Ideal Heat Flow Source/LConn1
  Ideal Heat Flow Source/RConn1 -- P_in/RConn1

== system Application_Problem_Solution/Battery7/Thermal Model ==
  Battery thermal mass : fl_lib/Thermal/Thermal Elements/Thermal Mass  mass=cell_mass kg  sp_heat=cell_Cp_heat J/kg/K  T_specify=on  T_priority=High  T=T_init K  T_nominal_specify=off  T_nominal_unit=K  T_nominal_value=1  Q_specify=off  Q_priority=High  Q=0 J/s  Q_nominal_specify=off  Q_nominal_unit=W  Q_nominal_value=1
  Ideal Temperature Sensor : fl_lib/Thermal/Thermal Sensors/Temperature Sensor
  Ideal Heat Flow Source : fl_lib/Thermal/Thermal Sources/Controlled Heat Flow Rate Source
      settings: SourceProductName=Simscape
  Thermal Reference1 : fl_lib/Thermal/Thermal Elements/Thermal Reference
  Thermal Reference2 : fl_lib/Thermal/Thermal Elements/Thermal Reference
  P_in : PMIOPort  Tag=PMCPort  Side=Left
  H : PMIOPort  Tag=PMCPort  Port=2  Side=Left
  T : PMIOPort  Tag=PMCPort  Port=3  Side=Right
  connections:
  Ideal Heat Flow Source/RConn1 -- P_in/RConn1
  Ideal Heat Flow Source/LConn1 -- Battery thermal mass/LConn1 -- H/RConn1 -- Ideal Temperature Sensor/LConn1
  Thermal Reference1/LConn1 -- Ideal Heat Flow Source/RConn2
  Ideal Temperature Sensor/RConn2 -- T/RConn1
  Thermal Reference2/LConn1 -- Ideal Temperature Sensor/RConn1

== system Application_Problem_Solution/Battery8/Thermal Model ==
  Battery thermal mass : fl_lib/Thermal/Thermal Elements/Thermal Mass  mass=cell_mass kg  sp_heat=cell_Cp_heat J/kg/K  T_specify=on  T_priority=High  T=T_init K  T_nominal_specify=off  T_nominal_unit=K  T_nominal_value=1  Q_specify=off  Q_priority=High  Q=0 J/s  Q_nominal_specify=off  Q_nominal_unit=W  Q_nominal_value=1
  Ideal Temperature Sensor : fl_lib/Thermal/Thermal Sensors/Temperature Sensor
  Ideal Heat Flow Source : fl_lib/Thermal/Thermal Sources/Controlled Heat Flow Rate Source
      settings: SourceProductName=Simscape
  Thermal Reference1 : fl_lib/Thermal/Thermal Elements/Thermal Reference
  Thermal Reference2 : fl_lib/Thermal/Thermal Elements/Thermal Reference
  P_in : PMIOPort  Tag=PMCPort  Side=Left
  H : PMIOPort  Tag=PMCPort  Port=2  Side=Left
  T : PMIOPort  Tag=PMCPort  Port=3  Side=Right
  connections:
  Thermal Reference2/LConn1 -- Ideal Temperature Sensor/RConn1
  Ideal Temperature Sensor/RConn2 -- T/RConn1
  Thermal Reference1/LConn1 -- Ideal Heat Flow Source/RConn2
  Ideal Temperature Sensor/LConn1 -- H/RConn1 -- Battery thermal mass/LConn1 -- Ideal Heat Flow Source/LConn1
  Ideal Heat Flow Source/RConn1 -- P_in/RConn1

== system Application_Problem_Solution/Battery9/Thermal Model ==
  Battery thermal mass : fl_lib/Thermal/Thermal Elements/Thermal Mass  mass=cell_mass kg  sp_heat=cell_Cp_heat J/kg/K  T_specify=on  T_priority=High  T=T_init K  T_nominal_specify=off  T_nominal_unit=K  T_nominal_value=1  Q_specify=off  Q_priority=High  Q=0 J/s  Q_nominal_specify=off  Q_nominal_unit=W  Q_nominal_value=1
  Ideal Temperature Sensor : fl_lib/Thermal/Thermal Sensors/Temperature Sensor
  Ideal Heat Flow Source : fl_lib/Thermal/Thermal Sources/Controlled Heat Flow Rate Source
      settings: SourceProductName=Simscape
  Thermal Reference1 : fl_lib/Thermal/Thermal Elements/Thermal Reference
  Thermal Reference2 : fl_lib/Thermal/Thermal Elements/Thermal Reference
  P_in : PMIOPort  Tag=PMCPort  Side=Left
  H : PMIOPort  Tag=PMCPort  Port=2  Side=Left
  T : PMIOPort  Tag=PMCPort  Port=3  Side=Right
  connections:
  Ideal Heat Flow Source/RConn1 -- P_in/RConn1
  Ideal Heat Flow Source/LConn1 -- Battery thermal mass/LConn1 -- H/RConn1 -- Ideal Temperature Sensor/LConn1
  Thermal Reference1/LConn1 -- Ideal Heat Flow Source/RConn2
  Ideal Temperature Sensor/RConn2 -- T/RConn1
  Thermal Reference2/LConn1 -- Ideal Temperature Sensor/RConn1
